simulink model "SimulinkModel"  (R2023b)
settings: Solver=FixedStepAuto  StartTime=0.0  StopTime=10.0  FixedStep=param.rateTransition_Main  RelTol=1e-3  EnableMultiTasking=on
undefined symbols (not defined in the file or in its folder): lidarMeasurement, param, SensorDataOS2, timestamp
libraries: simulink x30, GenericTarget x11, etargetslib x8
(part 3 of 3)

== matlab function SimulinkModel/Lidar Message/SendLidar/getNavMsg ==
  data: reset input; nodeID input; timestampUTC input double; navMsg input double; Lidar_ output Bus: busRawSensorMessage_LidarOdometry; numberDelay input; idx_ output uint32
function [Lidar_,idx_]  = getNavMsg(reset,nodeID,timestampUTC,navMsg,numberDelay)
    % input
    % navMsg:(23)
	% 1-sampletime
	% 2-timeStampUTC
	% 3-Lat
	% 4-Lon
	% 5-Alt
	% 6-Roll
	% 7-Pitch
	% 8-Yaw
	% 9-VelNorth
	% 10-VelEast
	% 11-VelDown
	% 12-VelU
	% 13-VelV
	% 14-VelW
	% 15-VelP
	% 16-VelQ
	% 17-VelR
	% 18-AccU
	% 19-AccV
	% 20-AccW
	% 21-AccP
	% 22-AccQ
	% 23-AccR

    % output
    % 1-Lidar
    % 2-index

    persistent origin; if(isempty(origin)), origin = zeros(1,10,'double'); end 
    persistent bufferInertialSample; if(isempty(bufferInertialSample)), bufferInertialSample = zeros(1,7,'double'); end
    persistent bufferOdomSample; if(isempty(bufferOdomSample)), bufferOdomSample = zeros(1,7,'double'); end
    persistent bufferSE3Sample; if(isempty(bufferSE3Sample)), bufferSE3Sample = eye(4); end
    persistent bufferSO3Sample; if(isempty(bufferSO3Sample)), bufferSO3Sample = eye(3); end
    persistent bufferTransSample; if(isempty(bufferTransSample)), bufferTransSample = zeros(3,1); end

    %persistent counter; if(isempty(counter)), counter = uint32(0); end

    interpolateComplete = false;
    eventReset = (reset > 0.0);
    Lidar_ = LOstruct();
    %Lidar2_ = LOstruct();


    if navMsg(2,1) <= timestampUTC && navMsg(2,numberDelay) >= timestampUTC
        %   interpolate
        [~,idx] = mink(abs(navMsg(2,:) - timestampUTC),2);
        timestamp = navMsg(2,:);
        intNavMsg = ( navMsg(:,idx(2)) - navMsg(:,idx(1)) ) ./ ( timestamp(1,idx(2)) - timestamp(1,idx(1)) ) .* ( timestampUTC - timestamp(1,idx(1)) ) + navMsg(:,idx(1));
        idx_ = uint32(idx(1));
        intNavMsg(2,1) = timestampUTC;
        interpolateComplete = true;

        % update valid
        Lidar_.valid = interpolateComplete;
    else
        idx_ = uint32(0);
        intNavMsg = zeros(23,1,'double');

        % update valid
        Lidar_.valid = interpolateComplete;
    end
    
    if interpolateComplete
        x = intNavMsg(6:8,1);
        y = SymmetricalAngle(x);
        intNavMsg(6:8,1) = y;
        roll = intNavMsg(6,1);
        pitch = intNavMsg(7,1);
        yaw = intNavMsg(8,1);
        q = getQuat(roll,pitch,yaw); % vector 4,1

        if eventReset

            origin = [intNavMsg(3),intNavMsg(4),intNavMsg(5),intNavMsg(6),intNavMsg(7),intNavMsg(8),q(1),q(2),q(3),q(4)];
            bufferInertialSample = [intNavMsg(2),intNavMsg(9),intNavMsg(10),intNavMsg(11),intNavMsg(15),intNavMsg(16),intNavMsg(17)];          % [timestamp,VelNorth,VelEast,VelDown,VelP,VelQ,VelR]
            % update navMeasurement
            [N,E,D] = ave.LLA2NED(intNavMsg(3),intNavMsg(4),intNavMsg(5),origin(1),origin(2),origin(3));
            bufferOdomSample = [N,E,D,q(1),q(2),q(3),q(4)];                                                                                     % [north,east,down,qw,qx,qy,qz]
            bufferSE3Sample = TransformMatrix(bufferOdomSample); % T12
            bufferSO3Sample = bufferSE3Sample(1:3,1:3);
            bufferTransSample = bufferSE3Sample(1:3,4);
            
            % update reset
            Lidar_.reset = reset;

            % update origin
            Lidar_.origin = origin;
            
            % update timestamp
            Lidar_.timestamp.timestamp = intNavMsg(2);
            
            % ############################################################
            % lidar tweak output
            %Lidar2_ = Lidar_;
            % ############################################################

            % update counter
            % counter = uint32(1);
            
        else
            % update counter
            % counter = counter + uint32(1);

            % ############################################################
            % output for lidar groundtruth
            % ############################################################

            % update reset
            Lidar_.reset = reset;

            % update nodeID
            Lidar_.nodeID = nodeID;
            
            % update origin
            Lidar_.origin = origin;

            % update navMeasurement
            [N,E,D] = ave.LLA2NED(intNavMsg(3),intNavMsg(4),intNavMsg(5),origin(1),origin(2),origin(3));

            Lidar_.navMeasurement.latitude = intNavMsg(3);
            Lidar_.navMeasurement.longitude = intNavMsg(4);
            Lidar_.navMeasurement.altitude = intNavMsg(5);
            Lidar_.navMeasurement.north = N;
            Lidar_.navMeasurement.east = E;
            Lidar_.navMeasurement.down = D;
            Lidar_.navMeasurement.roll = intNavMsg(6);
            Lidar_.navMeasurement.pitch = intNavMsg(7);
            Lidar_.navMeasurement.yaw = intNavMsg(8);
            Lidar_.navMeasurement.qw = q(1);
            Lidar_.navMeasurement.qx = q(2);
            Lidar_.navMeasurement.qy = q(3);
            Lidar_.navMeasurement.qz = q(4);
            Lidar_.navMeasurement.velNorth = intNavMsg(9);
            Lidar_.navMeasurement.velEast = intNavMsg(10);
            Lidar_.navMeasurement.velDown = intNavMsg(11);
            Lidar_.navMeasurement.velU = intNavMsg(12);
            Lidar_.navMeasurement.velV = intNavMsg(13);
            Lidar_.navMeasurement.velW = intNavMsg(14);
            Lidar_.navMeasurement.velP = intNavMsg(15);
            Lidar_.navMeasurement.velQ = intNavMsg(16);
            Lidar_.navMeasurement.velR = intNavMsg(17);
            Lidar_.navMeasurement.accU = intNavMsg(18);
            Lidar_.navMeasurement.accV = intNavMsg(19);
            Lidar_.navMeasurement.accW = intNavMsg(20);
            Lidar_.navMeasurement.accP = intNavMsg(21);
            Lidar_.navMeasurement.accQ = intNavMsg(22);
            Lidar_.navMeasurement.accR = intNavMsg(23);

            % update CVCAMeasurement
            ts = intNavMsg(2) - bufferInertialSample(1);
            dR = expm(skew([bufferInertialSample(5),bufferInertialSample(6),bufferInertialSample(7)]) * ts);                         % change in rotation

            dN = bufferInertialSample(2) * ts;
            dE = bufferInertialSample(3) * ts;
            dD = bufferInertialSample(4) * ts; 
            dp = [dN,dE,dD]';

            % dT = eye(4);
            % dT(1:3,1:3) = dR;
            % dT(1:3,4) = dp;

            Cnew = bufferSO3Sample * dR;
            tnew = bufferTransSample + dp;
            
            %bufferSE3Sample= bufferSE3Sample * dT;

            %bufferSE3Sample(3,4) = bufferSE3Sample(3,4)/10; % To test: what happen if divide line 50 with 1000. (ans:=)

            % tnew = (bufferSE3Sample(1:3,4))';
            % Cnew = bufferSE3Sample(1:3,1:3);
            % tnew = bufferTransSample;
            % Cnew = bufferSO3Sample;
            [roll_, pitch_, yaw_] = EulerZYX(Cnew);
            quat = getQuat(roll_,pitch_,yaw_);

            bufferOdomSample = [tnew(1),tnew(2),tnew(3),quat(1),quat(2),quat(3),quat(4)];
            bufferSE3Sample = TransformMatrix(bufferOdomSample);
            bufferSO3Sample = bufferSE3Sample(1:3,1:3);
            bufferTransSample = bufferSE3Sample(1:3,4);

            [lat_,lon_,alt_] = ave.NED2LLA(tnew(1),tnew(2),tnew(3),origin(1),origin(2),origin(3));

            Lidar_.CVCAMeasurement.latitude = lat_;
            Lidar_.CVCAMeasurement.longitude = lon_;
            Lidar_.CVCAMeasurement.altitude = alt_;
            Lidar_.CVCAMeasurement.north = tnew(1);
            Lidar_.CVCAMeasurement.east = tnew(2);
            Lidar_.CVCAMeasurement.down = tnew(3);
            Lidar_.CVCAMeasurement.roll = roll_;
            Lidar_.CVCAMeasurement.pitch = pitch_;
            Lidar_.CVCAMeasurement.yaw = yaw_;
            Lidar_.CVCAMeasurement.qw = quat(1);
            Lidar_.CVCAMeasurement.qx = quat(2);
            Lidar_.CVCAMeasurement.qy = quat(3);
            Lidar_.CVCAMeasurement.qz = quat(4);

            % update timestamp
            Lidar_.timestamp.sampleTime = ts;
            Lidar_.timestamp.timestamp = intNavMsg(2);

             % update buffer inertial
            bufferInertialSample = [intNavMsg(2),intNavMsg(9),intNavMsg(10),intNavMsg(11),intNavMsg(15),intNavMsg(16),intNavMsg(17)];

        end
    end
end

function y = skew(u)
    y = [0 -u(3) u(2);
            u(3) 0 -u(1);
            -u(2) u(1) 0];
end

function [roll, pitch, yaw] = EulerZYX(R)
    %GenericINS.SensorFusion.EulerZYX Calculate the corresponding euler angles (zyx-convention) for a given rotation matrix (b-frame to n-frame).
    % 
    % PARAMETERS
    % R ... 3x3 Rotation matrix (b-frame to n-frame).
    % 
    % RETURN
    % roll  ... Resulting roll angle in radians.
    % pitch ... Resulting pitch angle in radians.
    % yaw   ... Resulting yaw angle in radians.
    R = reshape(R, [3 3]);
    roll = SymmetricalAngle(atan2(R(3,2), R(3,3)));
    pitch = -real(asin(min(max(R(3,1),-1.0),1.0)));
    yaw = SymmetricalAngle(atan2(R(2,1), R(1,1)));
end

function T = TransformMatrix(x)
    q = x(4:7);
    q = (reshape(q,1,4))';
    C = Cb2n(q);
    T = eye(4);
    T(1:3,1:3) = C;
    p = x(1:3);
    p = (reshape(p,1,3))';
    T(1:3,4) = p;
end

function C = Cb2n(q)
    %GenericINS.SensorFusion.Cb2n Calculate the rotation matrix for a given unit quaternion.
    % 
    % PARAMETERS
    % q ... 4x1 normalized unit quaternion (b-frame to n-frame).
    % 
    % RETURN
    % C ... 3x3 rotation matrix (b-frame to n-frame).
    q = reshape(q, [4 1]);
    q0q0 = q(1) * q(1);
    q1q1 = q(2) * q(2);
    q2q2 = q(3) * q(3);
    q3q3 = q(4) * q(4);
    q1q2 = q(2) * q(3);
    q0q3 = q(1) * q(4);
    q1q3 = q(2) * q(4);
    q0q2 = q(1) * q(3);
    q2q3 = q(3) * q(4);
    q0q1 = q(1) * q(2);
    C = [
        q0q0+q1q1-q2q2-q3q3 q1q2+q1q2-q0q3-q0q3 q1q3+q1q3+q0q2+q0q2;
        q1q2+q1q2+q0q3+q0q3 q0q0-q1q1+q2q2-q3q3 q2q3+q2q3-q0q1-q0q1;
        q1q3+q1q3-q0q2-q0q2 q2q3+q2q3+q0q1+q0q1 q0q0-q1q1-q2q2+q3q3;
    ];
end

function y = SymmetricalAngle(x)
    %GenericINS.SensorFusion.SymmetricalAngle Convert a given angle x [rad] to an output angle y [rad] with y being in range [-pi, +pi).
    % 
    % PARAMETERS
    % x ... Input angle in radians, either scalar or n-dimensional.
    % 
    % RETURN
    % y ... Output angle in radians being in range [-pi, pi).
    x = x - 6.28318530717959 * fix(x * 0.159154943091895);
    y = x + 6.28318530717959 * double(x < -3.14159265358979) - 6.28318530717959 * double(x >= 3.14159265358979);
end

function y = getQuat(roll,pitch,yaw)
    % roll pitch, yaw in radian
    phi = 0.5 * roll;
    theta = 0.5 * pitch;
    psi = 0.5 * yaw;
    
    c1 = cos(phi);
    c2 = cos(theta);
    c3 = cos(psi);
    s1 = sin(phi);
    s2 = sin(theta);
    s3 = sin(psi);
    
    % Quaternion [4,1] = [qw;qx;qy;qz]
    u = [c1*c2*c3 + s1*s2*s3; s1*c2*c3 - c1*s2*s3; c1*s2*c3 + s1*c2*s3; c1*c2*s3 - s1*s2*c3];
    y = Normalize(u);
end

function y = Normalize(u)
    % GenericINS.SensorFusion.Normalize Safe normalization.
    % 
    % PARAMETERS
    % u ... Input vector. Must contain at least one element!
    % 
    % RETURN
    % y ... Normalized output vector. If input vector is close to zero, a default vector will be returned.
    len = norm(u);
    if(len < 1e-12)
        u = zeros(size(u));
        u(1) = 1.0;
        len = 1.0;
    end
    y = (1.0 / len) * u;
end  

function mystruct = LOstruct()
%init value
    reset = 0;
    valid = false;
    nodeID = uint32(0);
    origin = zeros(1,10,'double');

    timestamp.timestamp = 0;            % double
    timestamp.timestampGT = 0;          % double
    timestamp.sampleTime = 0;           % double
    
    lidarMeasurement.numberPoint = uint32(0);                           % uint32
    lidarMeasurement.points = zeros(131072,3,'single');                 % single
    lidarMeasurement.pointsReflect = zeros(131072,3,'single');          % single
    lidarMeasurement.pointsTimestamp = zeros(131072,1,'double');        % double
    lidarMeasurement.pointsMeasurementID = zeros(131072,1,'single');    % single

    lidarMeasurement2.numberPoint = uint32(0);                           % uint32
    lidarMeasurement2.points = zeros(131072,3,'single');                 % single
    lidarMeasurement2.pointsReflect = zeros(131072,3,'single');          % single
    lidarMeasurement2.pointsTimestamp = zeros(131072,1,'double');        % double
    lidarMeasurement2.pointsMeasurementID = zeros(131072,1,'single');    % single
    
    navMeasurement.latitude = 0;            % double
    navMeasurement.longitude = 0;           % double
    navMeasurement.altitude = 0;            % double
    navMeasurement.north = 0;               % double
    navMeasurement.east = 0;                % double
    navMeasurement.down = 0;                % double
    navMeasurement.roll = 0;                % double
    navMeasurement.pitch = 0;               % double
    navMeasurement.yaw = 0;                 % double
    navMeasurement.qw = 0;                  % double
    navMeasurement.qx = 0;                  % double
    navMeasurement.qy = 0;                  % double
    navMeasurement.qz = 0;                  % double
    navMeasurement.velNorth = 0;            % double
    navMeasurement.velEast = 0;             % double
    navMeasurement.velDown = 0;             % double
    navMeasurement.velU = 0;                % double
    navMeasurement.velV = 0;                % double
    navMeasurement.velW = 0;                % double
    navMeasurement.velP = 0;                % double
    navMeasurement.velQ = 0;                % double
    navMeasurement.velR = 0;                % double
    navMeasurement.accU = 0;                % double
    navMeasurement.accV = 0;                % double
    navMeasurement.accW = 0;                % double
    navMeasurement.accP = 0;                % double
    navMeasurement.accQ = 0;                % double
    navMeasurement.accR = 0;                % double

    navMeasurementSD.stdLat = 1;            % double
    navMeasurementSD.stdLon = 1;           % double
    navMeasurementSD.stdAlt = 1;            % double
    navMeasurementSD.stdNorth = 1;               % double
    navMeasurementSD.stdEast = 1;                % double
    navMeasurementSD.stdDown = 1;                % double
    navMeasurementSD.stdRoll = 1;                % double
    navMeasurementSD.stdPitch = 1;               % double
    navMeasurementSD.stdYaw = 1;                 % double
    navMeasurementSD.stdQw = 1;                  % double
    navMeasurementSD.stdQx = 1;                  % double
    navMeasurementSD.stdQy = 1;                  % double
    navMeasurementSD.stdQz = 1;                  % double
    navMeasurementSD.stdVelNorth = 1;            % double
    navMeasurementSD.stdVelEast = 1;             % double
    navMeasurementSD.stdVelDown = 1;             % double
    navMeasurementSD.stdVelU = 1;                % double
    navMeasurementSD.stdVelV = 1;                % double
    navMeasurementSD.stdVelW = 1;                % double
    navMeasurementSD.stdVelP = 1;                % double
    navMeasurementSD.stdVelQ = 1;                % double
    navMeasurementSD.stdVelR = 1;                % double
    navMeasurementSD.stdAccU = 1;                % double
    navMeasurementSD.stdAccV = 1;                % double
    navMeasurementSD.stdAccW = 1;                % double
    navMeasurementSD.stdAccP = 1;                % double
    navMeasurementSD.stdAccQ = 1;                % double
    navMeasurementSD.stdAccR = 1;                % double

    CVCAMeasurement.latitude = 0;            % double
    CVCAMeasurement.longitude = 0;           % double
    CVCAMeasurement.altitude = 0;            % double
    CVCAMeasurement.north = 0;               % double
    CVCAMeasurement.east = 0;                % double
    CVCAMeasurement.down = 0;                % double
    CVCAMeasurement.roll = 0;                % double
    CVCAMeasurement.pitch = 0;               % double
    CVCAMeasurement.yaw = 0;                 % double
    CVCAMeasurement.qw = 0;                  % double
    CVCAMeasurement.qx = 0;                  % double
    CVCAMeasurement.qy = 0;                  % doubleCVCAMeasurement
    CVCAMeasurement.qz = 0;                  % double
    CVCAMeasurement.velNorth = 0;            % double
    CVCAMeasurement.velEast = 0;             % double
    CVCAMeasurement.velDown = 0;             % double
    CVCAMeasurement.velU = 0;                % double
    CVCAMeasurement.velV = 0;                % double
    CVCAMeasurement.velW = 0;                % double
    CVCAMeasurement.velP = 0;                % double
    CVCAMeasurement.velQ = 0;                % double
    CVCAMeasurement.velR = 0;                % double
    CVCAMeasurement.accU = 0;                % double
    CVCAMeasurement.accV = 0;                % double
    CVCAMeasurement.accW = 0;                % double
    CVCAMeasurement.accP = 0;                % double
    CVCAMeasurement.accQ = 0;                % double
    CVCAMeasurement.accR = 0;                % double

    CVCAMeasurementSD.stdLat = 1;            % double
    CVCAMeasurementSD.stdLon = 1;           % double
    CVCAMeasurementSD.stdAlt = 1;            % double
    CVCAMeasurementSD.stdNorth = 1;               % double
    CVCAMeasurementSD.stdEast = 1;                % double
    CVCAMeasurementSD.stdDown = 1;                % double
    CVCAMeasurementSD.stdRoll = 1;                % double
    CVCAMeasurementSD.stdPitch = 1;               % double
    CVCAMeasurementSD.stdYaw = 1;                 % double
    CVCAMeasurementSD.stdQw = 1;                  % double
    CVCAMeasurementSD.stdQx = 1;                  % double
    CVCAMeasurementSD.stdQy = 1;                  % double
    CVCAMeasurementSD.stdQz = 1;                  % double
    CVCAMeasurementSD.stdVelNorth = 1;            % double
    CVCAMeasurementSD.stdVelEast = 1;             % double
    CVCAMeasurementSD.stdVelDown = 1;             % double
    CVCAMeasurementSD.stdVelU = 1;                % double
    CVCAMeasurementSD.stdVelV = 1;                % double
    CVCAMeasurementSD.stdVelW = 1;                % double
    CVCAMeasurementSD.stdVelP = 1;                % double
    CVCAMeasurementSD.stdVelQ = 1;                % double
    CVCAMeasurementSD.stdVelR = 1;                % double
    CVCAMeasurementSD.stdAccU = 1;                % double
    CVCAMeasurementSD.stdAccV = 1;                % double
    CVCAMeasurementSD.stdAccW = 1;                % double
    CVCAMeasurementSD.stdAccP = 1;                % double
    CVCAMeasurementSD.stdAccQ = 1;                % double
    CVCAMeasurementSD.stdAccR = 1;                % double

    LOMeasurement.latitude = 0;            % double
    LOMeasurement.longitude = 0;           % double
    LOMeasurement.altitude = 0;            % double
    LOMeasurement.north = 0;               % double
    LOMeasurement.east = 0;                % double
    LOMeasurement.down = 0;                % double
    LOMeasurement.roll = 0;                % double
    LOMeasurement.pitch = 0;               % double
    LOMeasurement.yaw = 0;                 % double
    LOMeasurement.qw = 0;                  % double
    LOMeasurement.qx = 0;                  % double
    LOMeasurement.qy = 0;                  % doubleCVCAMeasurement
    LOMeasurement.qz = 0;                  % double
    LOMeasurement.velNorth = 0;            % double
    LOMeasurement.velEast = 0;             % double
    LOMeasurement.velDown = 0;             % double
    LOMeasurement.velU = 0;                % double
    LOMeasurement.velV = 0;                % double
    LOMeasurement.velW = 0;                % double
    LOMeasurement.velP = 0;                % double
    LOMeasurement.velQ = 0;                % double
    LOMeasurement.velR = 0;                % double
    LOMeasurement.accU = 0;                % double
    LOMeasurement.accV = 0;                % double
    LOMeasurement.accW = 0;                % double
    LOMeasurement.accP = 0;                % double
    LOMeasurement.accQ = 0;                % double
    LOMeasurement.accR = 0;                % double

    LOMeasurementSD.stdLat = 1;            % double
    LOMeasurementSD.stdLon = 1;           % double
    LOMeasurementSD.stdAlt = 1;            % double
    LOMeasurementSD.stdNorth = 1;               % double
    LOMeasurementSD.stdEast = 1;                % double
    LOMeasurementSD.stdDown = 1;                % double
    LOMeasurementSD.stdRoll = 1;                % double
    LOMeasurementSD.stdPitch = 1;               % double
    LOMeasurementSD.stdYaw = 1;                 % double
    LOMeasurementSD.stdQw = 1;                  % double
    LOMeasurementSD.stdQx = 1;                  % double
    LOMeasurementSD.stdQy = 1;                  % double
    LOMeasurementSD.stdQz = 1;                  % double
    LOMeasurementSD.stdVelNorth = 1;            % double
    LOMeasurementSD.stdVelEast = 1;             % double
    LOMeasurementSD.stdVelDown = 1;             % double
    LOMeasurementSD.stdVelU = 1;                % double
    LOMeasurementSD.stdVelV = 1;                % double
    LOMeasurementSD.stdVelW = 1;                % double
    LOMeasurementSD.stdVelP = 1;                % double
    LOMeasurementSD.stdVelQ = 1;                % double
    LOMeasurementSD.stdVelR = 1;                % double
    LOMeasurementSD.stdAccU = 1;                % double
    LOMeasurementSD.stdAccV = 1;                % double
    LOMeasurementSD.stdAccW = 1;                % double
    LOMeasurementSD.stdAccP = 1;                % double
    LOMeasurementSD.stdAccQ = 1;                % double
    LOMeasurementSD.stdAccR = 1;                % double

    mystruct = struct('reset',reset,'valid',valid,'nodeID',nodeID,'origin',origin,'timestamp',timestamp,...
        'lidarMeasurement',lidarMeasurement,'lidarMeasurement2',lidarMeasurement2,...
        'navMeasurement',navMeasurement,'navMeasurementSD',navMeasurementSD,...
        'CVCAMeasurement',CVCAMeasurement,'CVCAMeasurementSD',CVCAMeasurementSD,...
        'LOMeasurement',LOMeasurement,'LOMeasurementSD',LOMeasurementSD);
end
